simulink model "robocup_model"  (Simulink 8.4)
settings: Solver=ode45  StartTime=0.0  StopTime=100.0  RelTol=1e-3
libraries: simulink x1

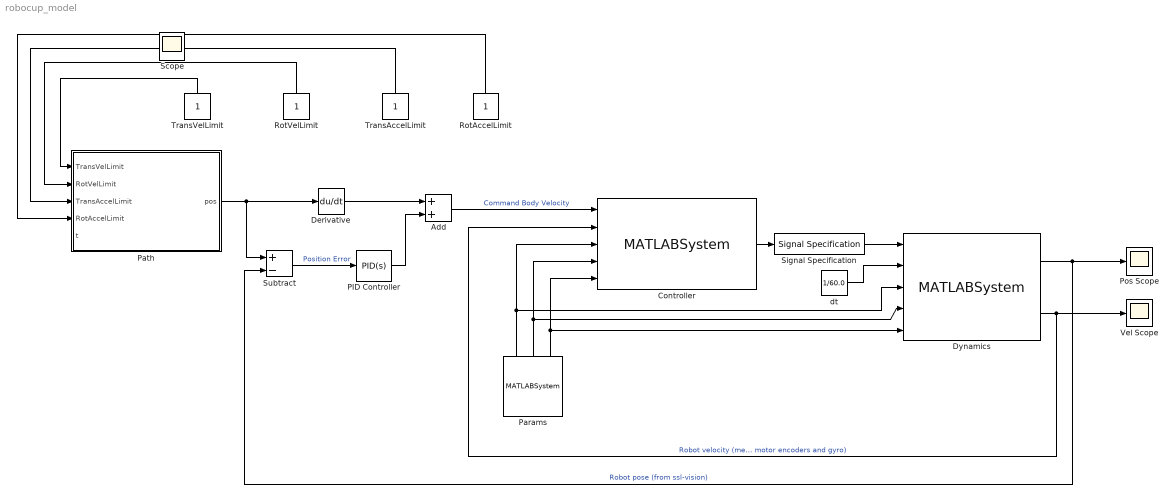
== system robocup_model ==
  Add : Sum
  Controller : MATLABSystem  System=RobotLqt  SimulateUsing=Interpreted execution  trans_vel_weight=1  rot_vel_weight=1  u_weight=1
  Derivative : Derivative
  Dynamics : MATLABSystem  System=Robot  SimulateUsing=Interpreted execution
  PID Controller : simulink/Continuous/PID Controller  Controller=PID  TimeDomain=Continuous-time  SampleTime=-1  IntegratorMethod=Forward Euler  FilterMethod=Forward Euler  Form=Parallel  P=1  I=1  D=0  N=100  InitialConditionSource=internal  InitialConditionForIntegrator=0  InitialConditionForFilter=0  ExternalReset=none  LimitOutput=off  UpperSaturationLimit=inf  LowerSaturationLimit=-inf  LinearizeAsGain=on  AntiWindupMode=none  Kb=1  TrackingMode=off  Kt=1  PParamMin=[]  PParamMax=[]  IParamMin=[]  IParamMax=[]  DParamMin=[]  DParamMax=[]  NParamMin=[]  NParamMax=[]  KbParamMin=[]  KbParamMax=[]  KtParamMin=[]  KtParamMax=[]  POutMin=[]  POutMax=[]  IOutMin=[]  IOutMax=[]  DOutMin=[]  DOutMax=[]  NOutMin=[]  NOutMax=[]  KbOutMin=[]  KbOutMax=[]  KtOutMin=[]  KtOutMax=[]  IntegratorOutMin=[]  IntegratorOutMax=[]  FilterOutMin=[]  FilterOutMax=[]  SumOutMin=[]  SumOutMax=[]  SumI1OutMin=[]  SumI1OutMax=[]  SumI2OutMin=[]  SumI2OutMax=[]  SumI3OutMin=[]  SumI3OutMax=[]  SumDOutMin=[]  SumDOutMax=[]  SaturationOutMin=[]  SaturationOutMax=[]  IntegratorContinuousStateAttributes=''  IntegratorStateMustResolveToSignalObject=off  IntegratorRTWStateStorageClass=Auto  FilterContinuousStateAttributes=''  FilterStateMustResolveToSignalObject=off  FilterRTWStateStorageClass=Auto  DifferentiatorICPrevScaledInput=0  DifferentiatorOutMin=[]  DifferentiatorOutMax=[]  UseFilter=on
  Params : MATLABSystem  System=RobotParams  M_bot=1  I_bot=1  g=2.0/7.0  r=1  L=0.1  K_e=1  K_t=1  K_f=1  I_asm=1  V=1  wheel_angles=(pi/4 + (pi/2)*(0:3))'
  Path : MATLAB Function  TreatAsAtomicUnit=on
  Pos Scope : Scope
  RotAccelLimit : Constant
  RotVelLimit : Constant
  Signal Specification : SignalSpecification  OutDataTypeStr=double  Dimensions=[4 1]
  Subtract : Sum  Inputs=+-
  TransAccelLimit : Constant
  TransVelLimit : Constant
  Vel Scope : Scope
  dt : Constant  Value=1/60.0
  Scope : Scope
  wires:
  PID Controller/1 -> Add/2
  Derivative/1 -> Add/1
  Path/1(pos) -> Subtract/1, Derivative/1
  Subtract/1 -> PID Controller/1  "Position Error"
  Add/1 -> Controller/1  "Command Body Velocity"
  dt/1 -> Dynamics/2
  Params/1 -> Controller/3, Dynamics/3
  Params/2 -> Controller/4, Dynamics/4
  Params/3 -> Controller/5, Dynamics/5
  Dynamics/1 -> Pos Scope/1, Subtract/2  "Robot pose (from ssl-vision)"
  Dynamics/2 -> Controller/2, Vel Scope/1  "Robot velocity (measured from motor encoders and gyro)"
  TransVelLimit/1 -> Path/1(TransVelLimit)
  RotVelLimit/1 -> Path/2(RotVelLimit)
  TransAccelLimit/1 -> Path/3(TransAccelLimit)
  RotAccelLimit/1 -> Path/4(RotAccelLimit)
  Controller/1 -> Signal Specification/1
  Signal Specification/1 -> Dynamics/1

== matlab function Path ==
function pos = path(TransVelLimit, RotVelLimit, TransAccelLimit, RotAccelLimit, t)
%#codegen

pos = [0 0 0]';
